simulink model "fa_cosim"  (Simulink 7.8)
settings: Solver=ode23  StartTime=0.0  StopTime=0.1  RelTol=1e-3
model workspace (MAT data in the model file):
  DigitalFreq : Simulink.Parameter (value not decoded)
undefined symbols (not defined in the file or in its folder): a, b
libraries: simulink x3, modelsimlib x1
settings Model: Creator=obmun  LastModifiedBy=obmun  SimulationMode=accelerator

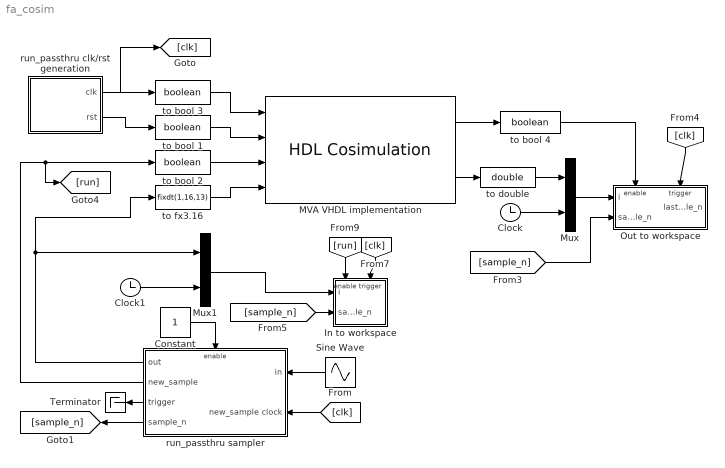
== system fa_cosim ==
  Clock : Clock
  Clock1 : Clock
  Constant : Constant
  In to workspace : Subsystem  TreatAsAtomicUnit=on
  MVA VHDL implementation : modelsimlib/HDL Cosimulation  PortPaths=/fa_cosim_wrapper/clk;/fa_cosim_wrapper/rst;/fa_cosim_wrapper/run_en;/fa_cosim_wrapper/run_passthru;/fa_cosim_wrapper/i;/fa_cosim_wrapper/o  PortModes=[1 1 1 2 1 2 ]  PortTimes=[-1,-1,-1,1/(2*DigitalFreq),-1,1/(2*DigitalFreq)]  PortSigns=[-1 -1 -1 -1 -1 1 ]  PortFracLengths=[0,0,0,0,0,13]  CommLocal=on  CommSharedMemory=on  CommPortNumber=4449  CommShowInfo=on  ClockModes=[]  ClockTimes=[]  TclPreSimCommand="puts \"Running Simulink Cosimulation block.\""  TclPostSimCommand="puts \"done\""  TimingMode=s  TimingScaleFactor=1  idxCellArray={'UNUSED_VAR'}  CosimBypass=Full Simulation  AllowDirectFeedthrough=off  ProductName=EDA Simulator Link MQ  RunAutoTimescale=off  HdlClocks=0
  Mux : Mux  Inputs=2
  Mux1 : Mux  Inputs=2
  Out to workspace : Subsystem  TreatAsAtomicUnit=on
  Sine Wave : Sin  Frequency=0*2*pi  Phase=pi/2  SampleTime=0
  Terminator : Terminator
  run_passthru clk/rst generation : Subsystem  mask{clk_f=DigitalFreq}
      mask prompts: clk_f "Clock frequency (Hz)"
      mask help:
      | Este bloque se encarga de generar una señal de reloj de frecuencia indicada
      | por el usuario mediante el parámetro correspondiente.
      | La salida reloj comienza en valor 0 y sube a 1 tras 1/2 del período espe-
      | cificado, generando el primer flanco ascendente.
      |
      | Desde el comienzo de la simulación hasta poco después de este primer flanco
      |  ascendente, mantiene la salida 'rst' a 1 para permitir situar en un esta-
      | do controlado aquellos bloques secuenciales que la señal de reloj controle.
      |
      | En bloques con reset de gran coste (como el bucle de amplitud del diseño
      | SPLL), es capaz de monitorizar la señal 'done' del bloque para controlar
      | cuando el procedimiento de reset llega a su fin. Mientras el reset tiene
      | lugar, la señal 'running' se mantendrá a 0. Una vez el reset ha finalizado,
      | running "sube" a 1.
      mask init:
      | rst_signal = [0, 1; 3/(4*clk_f), 0];
  run_passthru sampler : Subsystem  mask{f_s=1e4}
      mask prompts: f_s "Sample frequency (Hz)"
      mask help:
      | The "sampler" block is a LPF + S&H entity, a helper block for connecting
      | Simulink continuous signals to a VHDL block following the 'run_passthru' inter-
      | face specs.
      |
      | It takes care of antialias-filtering an input signal and sampling it, as
      | well of generating the 'run_en' for the VHDL block.
      |
      | Sampling freq. can be setup using the equivalente block parameter. Internal
      | LPF antialias freq is automatically adjusted. This block supposes a smpling
      | freq. low enough so the max(throughput, latency) of the block is lower than
      | the sampling period.
      |
      | An internal counter with current sample_n is maintained (starts at 0), and
      | sample_n is available as an output.
      |
      | ==== Input ports ====
      | == in ==
      | The values to be sampled. Can be a vector.
      |
      | == new_sample clock ==
      | Connect here the _digital_ clock used for driving the VHDL block. It's
      | required for correctly generating a just 1 cycle 'run' pulse for requesting
      | the begging of a new calculation to the connected 'run_done' interface.
      |
      | ==== Output ports ====
      | == out ==
      | The antialiased and held input vector
      |
      | == new_sample ==
      | This is the output for the 'run_en' signal generated by this block each time a
      | new sample is available.
      |
      | Each time a _new sample_ is available, a pulse of no more than 1 cycle of
      | 'new_sample clock' is generated.
      |
      | This pulse is generated the next rising edge after the new sample from 'in'
      |  signal has been taken, and it's delayed 1/4 of the new_sample clock. The
      | reason for this delay is to avoid problems inside the VHDL simulation when
      | the input signals rise at the _same_ exact time as the clock signal (which
      | we know it's not a sane way of doing things in the _real_ digital IC world).
      |
      | == trigger ==
      | This is a COPY of the internal trigger signal used to sample input value.
      |
      | == sample_n ==
      | Signal with the CURRENT sample number. The output of the internal sample counter. Type: integer.
      |
      | That is, before anything has been sampled, the output of this port is -1.
      | AFTER 1 sample is being hold, the ouput is 0, and so on.
      mask init:
      | [b, a] = sampler_block_init(gcb, f_s);
  to bool {1..4} (4 alike) : DataTypeConversion  OutDataTypeStr=boolean  RndMeth=Nearest  SaturateOnIntegerOverflow=on
  to double : DataTypeConversion  OutDataTypeStr=double
  to fx3.16 : DataTypeConversion  OutDataTypeStr=fixdt(1,16,13)  RndMeth=Nearest  SaturateOnIntegerOverflow=on
  wires:
  run_passthru clk/rst generation/1(clk) -> to bool 3/1, [clk]
  to bool 3/1 -> MVA VHDL implementation/1
  run_passthru clk/rst generation/2(rst) -> to bool 1/1
  to bool 1/1 -> MVA VHDL implementation/2
  to bool 2/1 -> MVA VHDL implementation/3
  run_passthru sampler/2(new_sample) -> to bool 2/1, [run]
  [clk] -> run_passthru sampler/2(new_sample clock)
  Sine Wave/1 -> run_passthru sampler/1(in)
  to fx3.16/1 -> MVA VHDL implementation/4
  run_passthru sampler/1(out) -> to fx3.16/1, Mux1/1
  Constant/1 -> run_passthru sampler/Enable
  run_passthru sampler/3(trigger) -> Terminator/1
  run_passthru sampler/4(sample_n) -> [sample_n]
  MVA VHDL implementation/2 -> to double/1
  to double/1 -> Mux/1
  Mux/1 -> Out to workspace/1(i)
  [sample_n] -> Out to workspace/2(sample_n)
  Clock/1 -> Mux/2
  MVA VHDL implementation/1 -> to bool 4/1
  to bool 4/1 -> Out to workspace/Enable
  [clk] -> Out to workspace/Trigger
  [sample_n] -> In to workspace/2(sample_n)
  Clock1/1 -> Mux1/2
  Mux1/1 -> In to workspace/1(i)
  [run] -> In to workspace/Enable
  [clk] -> In to workspace/Trigger

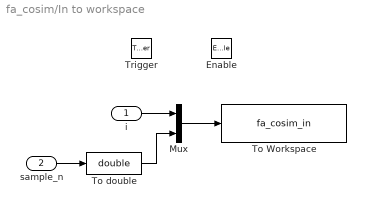
== system fa_cosim/In to workspace ==
  i : Inport
  sample_n : Inport  Port=2
  Enable : EnablePort
  Trigger : TriggerPort
  Mux : Mux  Inputs=2
  To Workspace : ToWorkspace  VariableName=fa_cosim_in  SampleTime=-1  SaveFormat=Array
  To double : DataTypeConversion  OutDataTypeStr=double
  wires:
  Mux/1 -> To Workspace/1
  i/1 -> Mux/1
  To double/1 -> Mux/2
  sample_n/1 -> To double/1

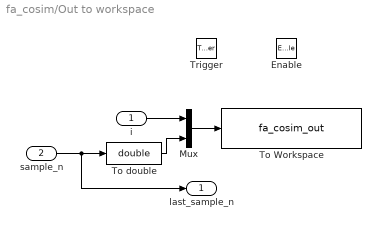
== system fa_cosim/Out to workspace ==
  i : Inport
  sample_n : Inport  Port=2
  Enable : EnablePort
  Trigger : TriggerPort  TriggerType=falling
  Mux : Mux  Inputs=2
  To Workspace : ToWorkspace  VariableName=fa_cosim_out  SampleTime=-1  SaveFormat=Array
  To double : DataTypeConversion  OutDataTypeStr=double
  last_sample_n : Outport  InitialOutput=-1
  wires:
  i/1 -> Mux/1
  Mux/1 -> To Workspace/1
  To double/1 -> Mux/2
  sample_n/1 -> To double/1, last_sample_n/1

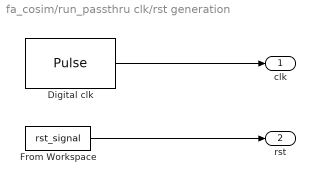
== system fa_cosim/run_passthru clk/rst generation ==
  Digital clk : DiscretePulseGenerator  Period=4  PulseWidth=2  PhaseDelay=2  SampleTime=1/(4*clk_f)
  From Workspace : FromWorkspace  VariableName=rst_signal  SampleTime=1/(4*clk_f)  Interpolate=off  OutputAfterFinalValue=Holding final value
  clk : Outport
  rst : Outport  Port=2
  wires:
  Digital clk/1 -> clk/1
  From Workspace/1 -> rst/1

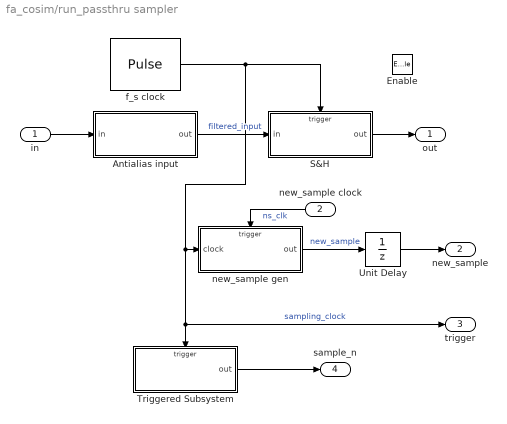
== system fa_cosim/run_passthru sampler ==
  in : Inport
  new_sample clock : Inport  Port=2
  Enable : EnablePort
  Antialias input : Subsystem  TreatAsAtomicUnit=on
  S&H : Subsystem  TreatAsAtomicUnit=on
  Triggered Subsystem : Subsystem  TreatAsAtomicUnit=on
  Unit Delay : UnitDelay  Description=|  SampleTime=-1
      | Esta ruta posee un sample rate dado por la señal de reloj (new_sample_clock).                                                                                                                                                                                                                                                                            
      |                                                                                                                                                                                                                                                                                                                                                          
      | Analicemos que valor tendrá aquí el "retardo unitario". Teniendo en cuenta la forma de generar el reloj digital de entrada por 'new_sample clock' que tenemos, el sampling rate en este bloque es de un sample cada 1/4 de período de señal de reloj de entrada por 'new_sample clock', es decir, la señal de reloj para los bloques cosimulados de VHDL.
      |                                                                                                                                                                                                                                                                                                                                                          
      | Por lo tanto, el retardo unitario será 1/4 de período del reloj digital externo.                                                                                                                                                                                                                                                                         
      |                                                                                                                                                                                                                                                                                                                                                          
      | La idea de introducir este retardo es para _evitar_ que la señal 'new_sample' suba y baje en el mismo instante de tiempo que el reloj digital al bloque VHDL. Así, al retrasarlo un 1/4 de ciclo de reloj, el bloque detectará la orden de 'sample' en el siguiente ciclo de reloj                                                                       
      |                                                                                                                                                                                                                                                                                                                                                          
      | De manera efectiva, este bloque retarda 1/4 de período de reloj la señal de sample.                                                                                                                                                                                                                                                                      
      |                                                                                                                                                                                                                                                                                                                                                          
      | El motivo: de lo contrario el SAMPLE sube a '1' _justo_ en el flanco ascendente de reloj de la PLL, y no nos interesan estasn coincidencias tan sutiles (recordemos las deltas en VHDL). Para que el sistema digital la coja, conviene retardarlo para que la orden de 'sample' sea enganchada en el siguiente ciclo de reloj digital
  f_s clock : DiscretePulseGenerator  Period=4  PulseWidth=2  PhaseDelay=1  SampleTime=1/(4*f_s)
  new_sample gen : Subsystem  TreatAsAtomicUnit=on
  out : Outport
  new_sample : Outport  Port=2  InitialOutput=0
  trigger : Outport  Port=3  InitialOutput=0
  sample_n : Outport  Port=4
  wires:
  in/1 -> Antialias input/1(in)
  S&H/1(out) -> out/1
  Antialias input/1(out) -> S&H/1(in)  "filtered_input"
  new_sample gen/1(out) -> Unit Delay/1  "new_sample"
  f_s clock/1 -> S&H/Trigger, new_sample gen/1(clock), trigger/1, Triggered Subsystem/Trigger  "sampling_clock"
  new_sample clock/1 -> new_sample gen/Trigger  "ns_clk"
  Unit Delay/1 -> new_sample/1
  Triggered Subsystem/1(out) -> sample_n/1

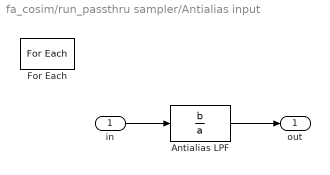
== system fa_cosim/run_passthru sampler/Antialias input ==
  in : Inport  Partition=on  PartitionDimension=1  PartitionWidth=1
  Antialias LPF : TransferFcn  Numerator=b  Denominator=a
  For Each : ForEach  DisableCoverage=on  IndexMode=One-based
  out : Outport  ConcatenationDimension=1
  wires:
  in/1 -> Antialias LPF/1
  Antialias LPF/1 -> out/1

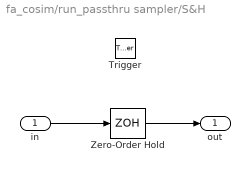
== system fa_cosim/run_passthru sampler/S&H ==
  in : Inport
  Trigger : TriggerPort
  Zero-Order Hold : ZeroOrderHold  SampleTime=-1
  out : Outport
  wires:
  in/1 -> Zero-Order Hold/1
  Zero-Order Hold/1 -> out/1

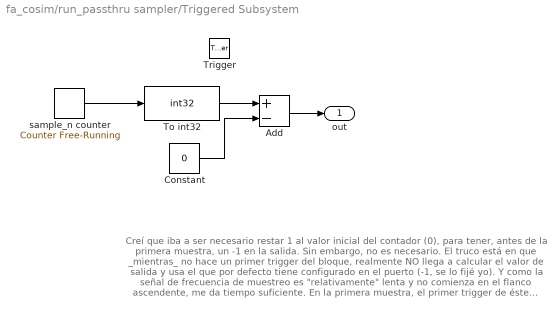
== system fa_cosim/run_passthru sampler/Triggered Subsystem ==
  note: Creí que iba a ser necesario restar 1 al valor inicial del contador (0), para tener, antes de la primera muestra, un -1 en la salida.
      | Sin embargo, no es necesario.
      | El truco está en que _mientras_ no hace un primer trigger del bloque, realmente NO llega a calcular el valor de salida y usa el que
      | por defecto tiene configurado en el puerto (-1, se lo fijé yo).
      | Y como la señal de frecuencia de muestreo es "relativamente" lenta y no comienza en el flanco ascendente, me da tiempo suficiente.
      |
      | En la primera muestra, el primer trigger de éste bloque y otros muchos, es el primer flanco ascendente, que lo que hace es inicializar el counter.
      | Entonces, en lugar de sacar 1, es la primera inicialización y sale un 0.
  Trigger : TriggerPort
  Add : Sum  Inputs=+-
  Constant : Constant  Value=0  OutDataTypeStr=int32
  To int32 : DataTypeConversion  OutDataTypeStr=int32
  sample_n counter : simulink/Sources/Counter Free-Running  NumBits=31  tsamp=-1
  out : Outport  InitialOutput=-1
  wires:
  sample_n counter/1 -> To int32/1
  To int32/1 -> Add/1
  Add/1 -> out/1
  Constant/1 -> Add/2

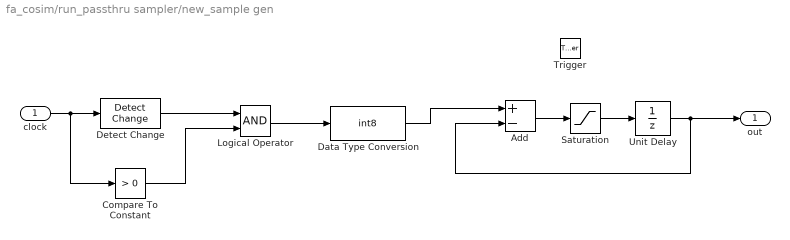
== system fa_cosim/run_passthru sampler/new_sample gen ==
  clock : Inport
  Trigger : TriggerPort
  Add : Sum  Inputs=+-
  Compare To Constant : simulink/Logic and Bit Operations/Compare To Constant  relop=>  const=0  OutDataTypeStr=boolean
  Data Type Conversion : DataTypeConversion  OutDataTypeStr=int8
  Detect Change : simulink/Logic and Bit Operations/Detect Change  vinit=0  InputProcessing=Inherited  OutDataTypeStr=boolean
  Logical Operator : Logic  AllPortsSameDT=off  OutDataTypeStr=boolean
  Saturation : Saturate  UpperLimit=1  LowerLimit=0
  Unit Delay : UnitDelay  SampleTime=-1
  out : Outport  InitialOutput=0
  wires:
  clock/1 -> Detect Change/1, Compare To Constant/1
  Unit Delay/1 -> Add/2, out/1
  Detect Change/1 -> Logical Operator/1
  Logical Operator/1 -> Data Type Conversion/1
  Data Type Conversion/1 -> Add/1
  Add/1 -> Saturation/1
  Saturation/1 -> Unit Delay/1
  Compare To Constant/1 -> Logical Operator/2
